simulink model "automata_learning"  (R2022a)
(part 8 of 10)

0.08787597715854645) + 1.0) - 1.0845412015914917 * (exp(0.37980449199676514 * x1 + 0.024216489866375923 * x2 - 1.1773580312728882) - 1.0) / (exp(0.37980449199676514 * x1 + 0.024216489866375923 * x2 - 1.1773580312728882) + 1.0) + 0.3358796238899231 * (exp(0.5314127802848816 * x1 - 0.2048840969800949 * x2 + 0.39898842573165894) - 1.0) / (exp(0.5314127802848816 * x1 - 0.2048840969800949 * x2 + 0.39898842573165894) + 1.0) - 0.04169782996177673 * (exp(0.9354951977729797 * x1 - 0.07700472325086594 * x2 + 1.2497409582138062) - 1.0) / (exp(0.9354951977729797 * x1 - 0.07700472325086594 * x2 + 1.2497409582138062) + 1.0) - 0.11417466402053833 * (exp(0.10226675122976303 * x1 + 0.7963433265686035 * x2 + 0.017623750492930412) - 1.0) / (exp(0.10226675122976303 * x1 + 0.7963433265686035 * x2 + 0.017623750492930412) + 1.0) + 0.7696085572242737 * (exp(0.7955979108810425 * x1 - 0.687153160572052 * x2 + 0.08714613318443298) - 1.0) / (exp(0.7955979108810425 * x1 - 0.687153160572052 * x2 + 0.08714613318443298) + 1.0) + 0.6961290836334229 * (exp(0.26372236013412476 * x1 + 0.9210137128829956 * x2 + 0.09220457822084427) - 1.0) / (exp(0.26372236013412476 * x1 + 0.9210137128829956 * x2 + 0.09220457822084427) + 1.0) + 0.7139140367507935 * (exp(0.48496493697166443 * x1 - 0.06392626464366913 * x2 + 0.7109420895576477) - 1.0) / (exp(0.48496493697166443 * x1 - 0.06392626464366913 * x2 + 0.7109420895576477) + 1.0) + 0.6749736666679382 * (exp(0.1728687733411789 * x1 + 0.6241433024406433 * x2 - 0.060625746846199036) - 1.0) / (exp(0.1728687733411789 * x1 + 0.6241433024406433 * x2 - 0.060625746846199036) + 1.0) - 0.7668593525886536 * (exp(1.1944445371627808 * x2 - 0.4847510755062103 * x1 + 0.370664119720459) - 1.0) / (exp(1.1944445371627808 * x2 - 0.4847510755062103 * x1 + 0.370664119720459) + 1.0) + 0.1648797243833542 * (exp(0.8625351190567017 * x1 + 1.135382890701294 * x2 + 0.11095273494720459) - 1.0) / (exp(0.8625351190567017 * x1 + 1.135382890701294 * x2 + 0.11095273494720459) + 1.0) + 0.4602258801460266 * (exp(0.7889838814735413 * x1 - 0.7123283743858337 * x2 + 0.2186594158411026) - 1.0) / (exp(0.7889838814735413 * x1 - 0.7123283743858337 * x2 + 0.2186594158411026) + 1.0) + 0.7145662903785706 * (exp(0.7569382190704346 * x1 + 0.9569622874259949 * x2 + 0.10968542098999023) - 1.0) / (exp(0.7569382190704346 * x1 + 0.9569622874259949 * x2 + 0.10968542098999023) + 1.0) + 0.519225537776947 * (exp(0.42037898302078247 * x1 + 0.8995851874351501 * x2 - 0.05327621474862099) - 1.0) / (exp(0.42037898302078247 * x1 + 0.8995851874351501 * x2 - 0.05327621474862099) + 1.0) - 0.04238021746277809) + 1.0) + 0.4274286925792694 * (exp(0.535226583480835 * (exp(1.2010539770126343 * x1 + 0.5278534889221191 * x2 + 0.1443147361278534) - 1.0) / (exp(1.2010539770126343 * x1 + 0.5278534889221191 * x2 + 0.1443147361278534) + 1.0) + 0.33181411027908325 * (exp(0.6581081748008728 * x2 - 0.0744652971625328 * x1 + 0.2685427665710449) - 1.0) / (exp(0.6581081748008728 * x2 - 0.0744652971625328 * x1 + 0.2685427665710449) + 1.0) + 0.48698070645332336 * (exp(0.6841858625411987 * x2 - 0.14291265606880188 * x1 + 0.28036966919898987) - 1.0) / (exp(0.6841858625411987 * x2 - 0.14291265606880188 * x1 + 0.28036966919898987) + 1.0) - 0.09695582091808319 * (exp(0.08600625395774841 * x1 + 0.6651319861412048 * x2 + 0.2726123034954071) - 1.0) / (exp(0.08600625395774841 * x1 + 0.6651319861412048 * x2 + 0.2726123034954071) + 1.0) + 0.6606088280677795 * (exp(0.42185717821121216 * x1 + 1.0105466842651367 * x2 + 0.3048625886440277) - 1.0) / (exp(0.42185717821121216 * x1 + 1.0105466842651367 * x2 + 0.3048625886440277) + 1.0) + 0.8615267276763916 * (exp(1.0305486917495728 * x1 - 0.22373104095458984 * x2 + 0.16078878939151764) - 1.0) / (exp(1.0305486917495728 * x1 - 0.22373104095458984 * x2 + 0.16078878939151764) + 1.0) - 0.5408587455749512 * (exp(0.27229365706443787 * x1 + 0.8539087772369385 * x2 - 0.08787597715854645) - 1.0) / (exp(0.27229365706443787 * x1 + 0.8539087772369385 * x2 - 0.08787597715854645) + 1.0) - 0.20088596642017365 * (exp(0.37980449199676514 * x1 + 0.024216489866375923 * x2 - 1.1773580312728882) - 1.0) / (exp(0.37980449199676514 * x1 + 0.024216489866375923 * x2 - 1.1773580312728882) + 1.0) + 0.5829349160194397 * (exp(0.5314127802848816 * x1 - 0.2048840969800949 * x2 + 0.39898842573165894) - 1.0) / (exp(0.5314127802848816 * x1 - 0.2048840969800949 * x2 + 0.39898842573165894) + 1.0) + 0.06516198068857193 * (exp(0.9354951977729797 * x1 - 0.07700472325086594 * x2 + 1.2497409582138062) - 1.0) / (exp(0.9354951977729797 * x1 - 0.07700472325086594 * x2 + 1.2497409582138062) + 1.0) + 0.28207874298095703 * (exp(0.10226675122976303 * x1 + 0.7963433265686035 * x2 + 0.017623750492930412) - 1.0) / (exp(0.10226675122976303 * x1 + 0.7963433265686035 * x2 + 0.017623750492930412) + 1.0) + 0.2900735139846802 * (exp(0.7955979108810425 * x1 - 0.687153160572052 * x2 + 0.08714613318443298) - 1.0) / (exp(0.7955979108810425 * x1 - 0.687153160572052 * x2 + 0.08714613318443298) + 1.0) - 0.3813025653362274 * (exp(0.26372236013412476 * x1 + 0.9210137128829956 * x2 + 0.09220457822084427) - 1.0) / (exp(0.26372236013412476 * x1 + 0.9210137128829956 * x2 + 0.09220457822084427) + 1.0) + 0.7694980502128601 * (exp(0.48496493697166443 * x1 - 0.06392626464366913 * x2 + 0.7109420895576477) - 1.0) / (exp(0.48496493697166443 * x1 - 0.06392626464366913 * x2 + 0.7109420895576477) + 1.0) + 0.11893359571695328 * (exp(0.1728687733411789 * x1 + 0.6241433024406433 * x2 - 0.060625746846199036) - 1.0) / (exp(0.1728687733411789 * x1 + 0.6241433024406433 * x2 - 0.060625746846199036) + 1.0) + 0.5006242394447327 * (exp(1.1944445371627808 * x2 - 0.4847510755062103 * x1 + 0.370664119720459) - 1.0) / (exp(1.1944445371627808 * x2 - 0.4847510755062103 * x1 + 0.370664119720459) + 1.0) + 0.3724484145641327 * (exp(0.8625351190567017 * x1 + 1.135382890701294 * x2 + 0.11095273494720459) - 1.0) / (exp(0.8625351190567017 * x1 + 1.135382890701294 * x2 + 0.11095273494720459) + 1.0) + 0.5391538739204407 * (exp(0.7889838814735413 * x1 - 0.7123283743858337 * x2 + 0.2186594158411026) - 1.0) / (exp(0.7889838814735413 * x1 - 0.7123283743858337 * x2 + 0.2186594158411026) + 1.0) - 0.25172242522239685 * (exp(0.7569382190704346 * x1 + 0.9569622874259949 * x2 + 0.10968542098999023) - 1.0) / (exp(0.7569382190704346 * x1 + 0.9569622874259949 * x2 + 0.10968542098999023) + 1.0) - 0.390072762966156 * (exp(0.42037898302078247 * x1 + 0.8995851874351501 * x2 - 0.05327621474862099) - 1.0) / (exp(0.42037898302078247 * x1 + 0.8995851874351501 * x2 - 0.05327621474862099) + 1.0) + 0.12838393449783325) - 1.0) / (exp(0.535226583480835 * (exp(1.2010539770126343 * x1 + 0.5278534889221191 * x2 + 0.1443147361278534) - 1.0) / (exp(1.2010539770126343 * x1 + 0.5278534889221191 * x2 + 0.1443147361278534) + 1.0) + 0.33181411027908325 * (exp(0.6581081748008728 * x2 - 0.0744652971625328 * x1 + 0.2685427665710449) - 1.0) / (exp(0.6581081748008728 * x2 - 0.0744652971625328 * x1 + 0.2685427665710449) + 1.0) + 0.48698070645332336 * (exp(0.6841858625411987 * x2 - 0.14291265606880188 * x1 + 0.28036966919898987) - 1.0) / (exp(0.6841858625411987 * x2 - 0.14291265606880188 * x1 + 0.28036966919898987) + 1.0) - 0.09695582091808319 * (exp(0.08600625395774841 * x1 + 0.6651319861412048 * x2 + 0.2726123034954071) - 1.0) / (exp(0.08600625395774841 * x1 + 0.6651319861412048 * x2 + 0.2726123034954071) + 1.0) + 0.6606088280677795 * (exp(0.42185717821121216 * x1 + 1.0105466842651367 * x2 + 0.3048625886440277) - 1.0) / (exp(0.42185717821121216 * x1 + 1.0105466842651367 * x2 + 0.3048625886440277) + 1.0) + 0.8615267276763916 * (exp(1.0305486917495728 * x1 - 0.22373104095458984 * x2 + 0.16078878939151764) - 1.0) / (exp(1.0305486917495728 * x1 - 0.22373104095458984 * x2 + 0.16078878939151764) + 1.0) - 0.5408587455749512 * (exp(0.27229365706443787 * x1 + 0.8539087772369385 * x2 - 0.08787597715854645) - 1.0) / (exp(0.27229365706443787 * x1 + 0.8539087772369385 * x2 - 0.08787597715854645) + 1.0) - 0.20088596642017365 * (exp(0.37980449199676514 * x1 + 0.024216489866375923 * x2 - 1.1773580312728882) - 1.0) / (exp(0.37980449199676514 * x1 + 0.024216489866375923 * x2 - 1.1773580312728882) + 1.0) + 0.5829349160194397 * (exp(0.5314127802848816 * x1 - 0.2048840969800949 * x2 + 0.39898842573165894) - 1.0) / (exp(0.5314127802848816 * x1 - 0.2048840969800949 * x2 + 0.39898842573165894) + 1.0) + 0.06516198068857193 * (exp(0.9354951977729797 * x1 - 0.07700472325086594 * x2 + 1.2497409582138062) - 1.0) / (exp(0.9354951977729797 * x1 - 0.07700472325086594 * x2 + 1.2497409582138062) + 1.0) + 0.28207874298095703 * (exp(0.10226675122976303 * x1 + 0.7963433265686035 * x2 + 0.017623750492930412) - 1.0) / (exp(0.10226675122976303 * x1 + 0.7963433265686035 * x2 + 0.017623750492930412) + 1.0) + 0.2900735139846802 * (exp(0.7955979108810425 * x1 - 0.687153160572052 * x2 + 0.08714613318443298) - 1.0) / (exp(0.7955979108810425 * x1 - 0.687153160572052 * x2 + 0.08714613318443298) + 1.0) - 0.3813025653362274 * (exp(0.26372236013412476 * x1 + 0.9210137128829956 * x2 + 0.09220457822084427) - 1.0) / (exp(0.26372236013412476 * x1 + 0.9210137128829956 * x2 + 0.09220457822084427) + 1.0) + 0.7694980502128601 * (exp(0.48496493697166443 * x1 - 0.06392626464366913 * x2 + 0.7109420895576477) - 1.0) / (exp(0.48496493697166443 * x1 - 0.06392626464366913 * x2 + 0.7109420895576477) + 1.0) + 0.11893359571695328 * (exp(0.1728687733411789 * x1 + 0.6241433024406433 * x2 - 0.060625746846199036) - 1.0) / (exp(0.1728687733411789 * x1 + 0.6241433024406433 * x2 - 0.060625746846199036) + 1.0) + 0.5006242394447327 * (exp(1.1944445371627808 * x2 - 0.4847510755062103 * x1 + 0.370664119720459) - 1.0) / (exp(1.1944445371627808 * x2 - 0.4847510755062103 * x1 + 0.370664119720459) + 1.0) + 0.3724484145641327 * (exp(0.8625351190567017 * x1 + 1.135382890701294 * x2 + 0.11095273494720459) - 1.0) / (exp(0.8625351190567017 * x1 + 1.135382890701294 * x2 + 0.11095273494720459) + 1.0) + 0.5391538739204407 * (exp(0.7889838814735413 * x1 - 0.7123283743858337 * x2 + 0.2186594158411026) - 1.0) / (exp(0.7889838814735413 * x1 - 0.7123283743858337 * x2 + 0.2186594158411026) + 1.0) - 0.25172242522239685 * (exp(0.7569382190704346 * x1 + 0.9569622874259949 * x2 + 0.10968542098999023) - 1.0) / (exp(0.7569382190704346 * x1 + 0.9569622874259949 * x2 + 0.10968542098999023) + 1.0) - 0.390072762966156 * (exp(0.42037898302078247 * x1 + 0.8995851874351501 * x2 - 0.05327621474862099) - 1.0) / (exp(0.42037898302078247 * x1 + 0.8995851874351501 * x2 - 0.05327621474862099) + 1.0) + 0.12838393449783325) + 1.0) + 0.16923418641090393 * (exp(0.8885021805763245 * (exp(1.2010539770126343 * x1 + 0.5278534889221191 * x2 + 0.1443147361278534) - 1.0) / (exp(1.2010539770126343 * x1 + 0.5278534889221191 * x2 + 0.1443147361278534) + 1.0) - 0.31739509105682373 * (exp(0.6581081748008728 * x2 - 0.0744652971625328 * x1 + 0.2685427665710449) - 1.0) / (exp(0.6581081748008728 * x2 - 0.0744652971625328 * x1 + 0.2685427665710449) + 1.0) + 0.4459865391254425 * (exp(0.6841858625411987 * x2 - 0.14291265606880188 * x1 + 0.28036966919898987) - 1.0) / (exp(0.6841858625411987 * x2 - 0.14291265606880188 * x1 + 0.28036966919898987) + 1.0) + 0.41351643204689026 * (exp(0.08600625395774841 * x1 + 0.6651319861412048 * x2 + 0.2726123034954071) - 1.0) / (exp(0.08600625395774841 * x1 + 0.6651319861412048 * x2 + 0.2726123034954071) + 1.0) + 0.13569283485412598 * (exp(0.42185717821121216 * x1 + 1.0105466842651367 * x2 + 0.3048625886440277) - 1.0) / (exp(0.42185717821121216 * x1 + 1.0105466842651367 * x2 + 0.3048625886440277) + 1.0) - 0.6290336847305298 * (exp(1.0305486917495728 * x1 - 0.22373104095458984 * x2 + 0.16078878939151764) - 1.0) / (exp(1.0305486917495728 * x1 - 0.22373104095458984 * x2 + 0.16078878939151764) + 1.0) - 0.06242078170180321 * (exp(0.27229365706443787 * x1 + 0.8539087772369385 * x2 - 0.08787597715854645) - 1.0) / (exp(0.27229365706443787 * x1 + 0.8539087772369385 * x2 - 0.08787597715854645) + 1.0) - 0.36062800884246826 * (exp(0.37980449199676514 * x1 + 0.024216489866375923 * x2 - 1.1773580312728882) - 1.0) / (exp(0.37980449199676514 * x1 + 0.024216489866375923 * x2 - 1.1773580312728882) + 1.0) - 0.22166602313518524 * (exp(0.5314127802848816 * x1 - 0.2048840969800949 * x2 + 0.39898842573165894) - 1.0) / (exp(0.5314127802848816 * x1 - 0.2048840969800949 * x2 + 0.39898842573165894) + 1.0) - 0.38659465312957764 * (exp(0.9354951977729797 * x1 - 0.07700472325086594 * x2 + 1.2497409582138062) - 1.0) / (exp(0.9354951977729797 * x1 - 0.07700472325086594 * x2 + 1.2497409582138062) + 1.0) + 0.017070304602384567 * (exp(0.10226675122976303 * x1 + 0.7963433265686035 * x2 + 0.017623750492930412) - 1.0) / (exp(0.10226675122976303 * x1 + 0.7963433265686035 * x2 + 0.017623750492930412) + 1.0) - 0.719062328338623 * (exp(0.7955979108810425 * x1 - 0.687153160572052 * x2 + 0.08714613318443298) - 1.0) / (exp(0.7955979108810425 * x1 - 0.687153160572052 * x2 + 0.08714613318443298) + 1.0) + 0.4505918323993683 * (exp(0.26372236013412476 * x1 + 0.9210137128829956 * x2 + 0.09220457822084427) - 1.0) / (exp(0.26372236013412476 * x1 + 0.9210137128829956 * x2 + 0.09220457822084427) + 1.0) + 0.02180497534573078 * (exp(0.48496493697166443 * x1 - 0.06392626464366913 * x2 + 0.7109420895576477) - 1.0) / (exp(0.48496493697166443 * x1 - 0.06392626464366913 * x2 + 0.7109420895576477) + 1.0) - 0.3865022361278534 * (exp(0.1728687733411789 * x1 + 0.6241433024406433 * x2 - 0.060625746846199036) - 1.0) / (exp(0.1728687733411789 * x1 + 0.6241433024406433 * x2 - 0.060625746846199036) + 1.0) + 0.8465549945831299 * (exp(1.1944445371627808 * x2 - 0.4847510755062103 * x1 + 0.370664119720459) - 1.0) / (exp(1.1944445371627808 * x2 - 0.4847510755062103 * x1 + 0.370664119720459) + 1.0) - 0.383506715297699 * (exp(0.8625351190567017 * x1 + 1.135382890701294 * x2 + 0.11095273494720459) - 1.0) / (exp(0.8625351190567017 * x1 + 1.135382890701294 * x2 + 0.11095273494720459) + 1.0) - 0.869685709476471 * (exp(0.7889838814735413 * x1 - 0.7123283743858337 * x2 + 0.2186594158411026) - 1.0) / (exp(0.7889838814735413 * x1 - 0.7123283743858337 * x2 + 0.2186594158411026) + 1.0) + 0.7902817130088806 * (exp(0.7569382190704346 * x1 + 0.9569622874259949 * x2 + 0.10968542098999023) - 1.0) / (exp(0.7569382190704346 * x1 + 0.9569622874259949 * x2 + 0.10968542098999023) + 1.0) + 0.506967306137085 * (exp(0.42037898302078247 * x1 + 0.8995851874351501 * x2 - 0.05327621474862099) - 1.0) / (exp(0.42037898302078247 * x1 + 0.8995851874351501 * x2 - 0.05327621474862099) + 1.0) + 0.11844814568758011) - 1.0) / (exp(0.8885021805763245 * (exp(1.2010539770126343 * x1 + 0.5278534889221191 * x2 + 0.1443147361278534) - 1.0) / (exp(1.2010539770126343 * x1 + 0.5278534889221191 * x2 + 0.1443147361278534) + 1.0) - 0.31739509105682373 * (exp(0.6581081748008728 * x2 - 0.0744652971625328 * x1 + 0.2685427665710449) - 1.0) / (exp(0.6581081748008728 * x2 - 0.0744652971625328 * x1 + 0.2685427665710449) + 1.0) + 0.4459865391254425 * (exp(0.6841858625411987 * x2 - 0.14291265606880188 * x1 + 0.28036966919898987) - 1.0) / (exp(0.6841858625411987 * x2 - 0.14291265606880188 * x1 + 0.28036966919898987) + 1.0) + 0.41351643204689026 * (exp(0.08600625395774841 * x1 + 0.6651319861412048 * x2 + 0.2726123034954071) - 1.0) / (exp(0.08600625395774841 * x1 + 0.6651319861412048 * x2 + 0.2726123034954071) + 1.0) + 0.13569283485412598 * (exp(0.42185717821121216 * x1 + 1.0105466842651367 * x2 + 0.3048625886440277) - 1.0) / (exp(0.42185717821121216 * x1 + 1.0105466842651367 * x2 + 0.3048625886440277) + 1.0) - 0.6290336847305298 * (exp(1.0305486917495728 * x1 - 0.22373104095458984 * x2 + 0.16078878939151764) - 1.0) / (exp(1.0305486917495728 * x1 - 0.22373104095458984 * x2 + 0.16078878939151764) + 1.0) - 0.06242078170180321 * (exp(0.27229365706443787 * x1 + 0.8539087772369385 * x2 - 0.08787597715854645) - 1.0) / (exp(0.27229365706443787 * x1 + 0.8539087772369385 * x2 - 0.08787597715854645) + 1.0) - 0.36062800884246826 * (exp(0.37980449199676514 * x1 + 0.024216489866375923 * x2 - 1.1773580312728882) - 1.0) / (exp(0.37980449199676514 * x1 + 0.024216489866375923 * x2 - 1.1773580312728882) + 1.0) - 0.22166602313518524 * (exp(0.5314127802848816 * x1 - 0.2048840969800949 * x2 + 0.39898842573165894) - 1.0) / (exp(0.5314127802848816 * x1 - 0.2048840969800949 * x2 + 0.39898842573165894) + 1.0) - 0.38659465312957764 * (exp(0.9354951977729797 * x1 - 0.07700472325086594 * x2 + 1.2497409582138062) - 1.0) / (exp(0.9354951977729797 * x1 - 0.07700472325086594 * x2 + 1.2497409582138062) + 1.0) + 0.017070304602384567 * (exp(0.10226675122976303 * x1 + 0.7963433265686035 * x2 + 0.017623750492930412) - 1.0) / (exp(0.10226675122976303 * x1 + 0.7963433265686035 * x2 + 0.017623750492930412) + 1.0) - 0.719062328338623 * (exp(0.7955979108810425 * x1 - 0.687153160572052 * x2 + 0.08714613318443298) - 1.0) / (exp(0.7955979108810425 * x1 - 0.687153160572052 * x2 + 0.08714613318443298) + 1.0) + 0.4505918323993683 * (exp(0.26372236013412476 * x1 + 0.9210137128829956 * x2 + 0.09220457822084427) - 1.0) / (exp(0.26372236013412476 * x1 + 0.9210137128829956 * x2 + 0.09220457822084427) + 1.0) + 0.02180497534573078 * (exp(0.48496493697166443 * x1 - 0.06392626464366913 * x2 + 0.7109420895576477) - 1.0) / (exp(0.48496493697166443 * x1 - 0.06392626464366913 * x2 + 0.7109420895576477) + 1.0) - 0.3865022361278534 * (exp(0.1728687733411789 * x1 + 0.6241433024406433 * x2 - 0.060625746846199036) - 1.0) / (exp(0.1728687733411789 * x1 + 0.6241433024406433 * x2 - 0.060625746846199036) + 1.0) + 0.8465549945831299 * (exp(1.1944445371627808 * x2 - 0.4847510755062103 * x1 + 0.370664119720459) - 1.0) / (exp(1.1944445371627808 * x2 - 0.4847510755062103 * x1 + 0.370664119720459) + 1.0) - 0.383506715297699 * (exp(0.8625351190567017 * x1 + 1.135382890701294 * x2 + 0.11095273494720459) - 1.0) / (exp(0.8625351190567017 * x1 + 1.135382890701294 * x2 + 0.11095273494720459) + 1.0) - 0.869685709476471 * (exp(0.7889838814735413 * x1 - 0.7123283743858337 * x2 + 0.2186594158411026) - 1.0) / (exp(0.7889838814735413 * x1 - 0.7123283743858337 * x2 + 0.2186594158411026) + 1.0) + 0.7902817130088806 * (exp(0.7569382190704346 * x1 + 0.9569622874259949 * x2 + 0.10968542098999023) - 1.0) / (exp(0.7569382190704346 * x1 + 0.9569622874259949 * x2 + 0.10968542098999023) + 1.0) + 0.506967306137085 * (exp(0.42037898302078247 * x1 + 0.8995851874351501 * x2 - 0.05327621474862099) - 1.0) / (exp(0.42037898302078247 * x1 + 0.8995851874351501 * x2 - 0.05327621474862099) + 1.0) + 0.11844814568758011) + 1.0) - 0.05044140666723251;
